simulink model "ex_separee_tf"  (R2019a)
settings: Solver=VariableStepAuto  StartTime=0.0  StopTime=10.0  RelTol=1e-3
values from neighbouring files (symbols this model uses):
  Bm = 1.074e-6    (= 1.074e-06)    [ex_separee.m]
  J = 0.21    [ex_separee.m]
  LAA = 0.01    [ex_separee.m]
  LAF = 0.004    [ex_separee.m]
  LFF = 0.167    [ex_separee.m]
  ra = 0.013    [ex_separee.m]
  rf = 1.43    [ex_separee.m]
  Tl = 2.493    [ex_separee.m]
  Va = 24    [ex_separee.m]
  Vf = 12    [ex_separee.m]
settings Model: Creator=azizi  LastModifiedBy=azizi

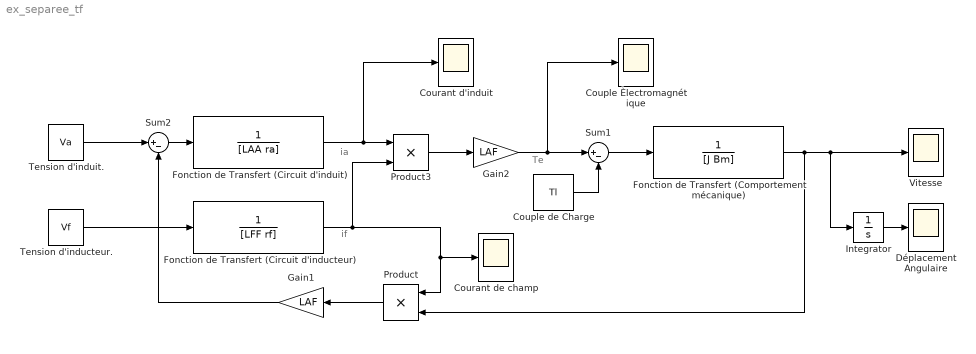
== system ex_separee_tf ==
  note: Te
  note: ia
  note: if
  "Couple de Charge " : Constant  Value=Tl
  Couple Èlectromagnétique : Scope
  Courant d'induit : Scope
  Courant de champ : Scope
  Déplacement Angulaire : Scope
  Fonction de Transfert (Circuit d'inducteur) : TransferFcn  Denominator=[LFF rf]
  Fonction de Transfert (Circuit d'induit) : TransferFcn  Denominator=[LAA ra]
  Fonction de Transfert (Comportement mécanique) : TransferFcn  Denominator=[J Bm]
  Gain1 : Gain  Gain=LAF
  Gain2 : Gain  Gain=LAF
  Integrator : Integrator
  Product : Product
  Product3 : Product
  Sum1 : Sum  Inputs=|+-
  Sum2 : Sum  Inputs=|+-
  "Tension d'inducteur. " : Constant  Value=Vf
  "Tension d'induit. " : Constant  Value=Va
  Vitesse : Scope
  wires:
  "Tension d'induit. "/1 -> Sum2/1
  Sum2/1 -> Fonction de Transfert (Circuit d'induit)/1
  Fonction de Transfert (Circuit d'induit)/1 -> Courant d'induit/1, Product3/1
  Fonction de Transfert (Circuit d'inducteur)/1 -> Product3/2, Product/1, Courant de champ/1
  Product/1 -> Gain1/1
  Gain1/1 -> Sum2/2
  Product3/1 -> Gain2/1
  Gain2/1 -> Sum1/1, Couple Èlectromagnétique/1
  Sum1/1 -> Fonction de Transfert (Comportement mécanique)/1
  Fonction de Transfert (Comportement mécanique)/1 -> Vitesse/1, Integrator/1, Product/2
  "Couple de Charge "/1 -> Sum1/2
  Integrator/1 -> Déplacement Angulaire/1
  "Tension d'inducteur. "/1 -> Fonction de Transfert (Circuit d'inducteur)/1
